simulink model "HeatExchanger"  (Simulink 8.3)
settings: Solver=ode4  StartTime=0.0  StopTime=800  FixedStep=.01  RelTol=1e-3
values from neighbouring files (symbols this model uses):
  delta_t = 0.5    [DoublePlant_STAT.mat]    (also in HeatExchanger_ps.m = 0.1; Initials.mat = 0.25; steady_state_data.mat = 0.1)
libraries: simulink x1
settings Model: Creator=Rhine  LastModifiedBy=wangwenchen
settings OptimizationCC: ExpressionDepthLimit=2147483647
settings DebuggingCC: FcnCallInpInsideContextMsg=UseLocalSettings

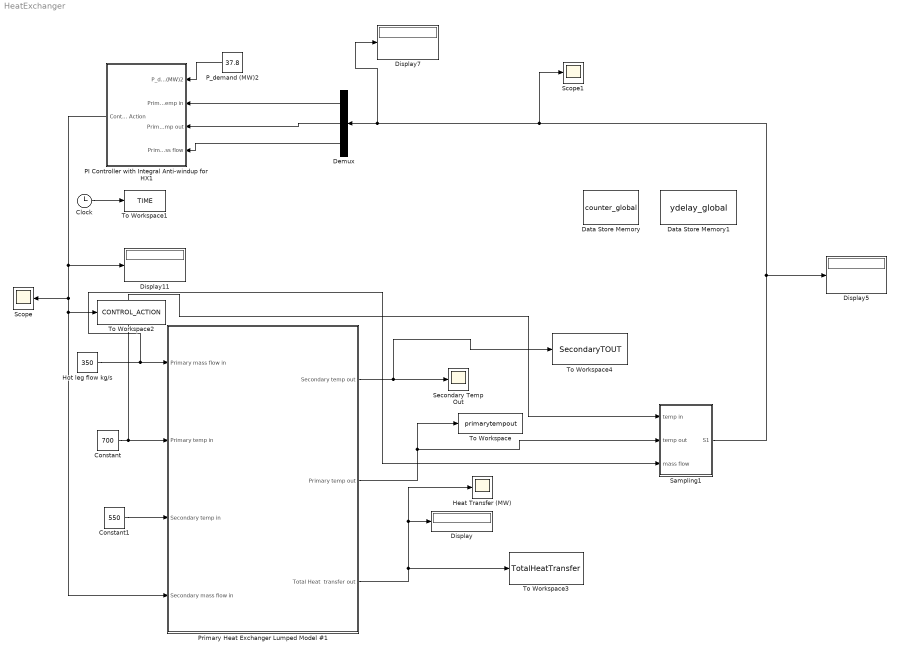
== system HeatExchanger ==
  Clock : Clock
  Constant : Constant  Value=700
  Constant1 : Constant  Value=550
  Data Store Memory : DataStoreMemory  DataStoreName=counter_global  ReadBeforeWriteMsg=warning  WriteAfterWriteMsg=warning  WriteAfterReadMsg=warning  OutDataTypeStr=int32
  Data Store Memory1 : DataStoreMemory  DataStoreName=ydelay_global  ReadBeforeWriteMsg=warning  WriteAfterWriteMsg=warning  WriteAfterReadMsg=warning  InitialValue=ones(10,1)  OutDataTypeStr=int32
  Demux : Demux  Outputs=3
  Display{,5,7,11} (4 alike) : Display
  Heat Transfer (MW) : Scope
      settings: TimeRange=30  YMin=23.3769  YMax=25.8377  SaveName=ScopeData3
  Hot leg flow kg/s : Constant  Value=350
  PI Controller with Integral Anti-windup for HX1 : Subsystem
  P_demand (MW)2 : Constant  Value=37.8
  Primary Heat Exchanger Lumped Model #1 : Subsystem
  Sampling1 : Subsystem
  Scope : Scope
      settings: SaveName=ScopeData2
  Scope1 : Scope
      settings: SaveName=ScopeData5
  Secondary Temp Out : Scope
      settings: YMin=639  YMax=640.4
  To Workspace : ToWorkspace  VariableName=primarytempout  SaveFormat=Timeseries  SampleTime=-1
  To Workspace1 : ToWorkspace  VariableName=TIME  SampleTime=-1
  To Workspace2 : ToWorkspace  VariableName=CONTROL_ACTION  SaveFormat=Timeseries  SampleTime=-1
  To Workspace3 : ToWorkspace  VariableName=TotalHeatTransfer  SaveFormat=Timeseries  SampleTime=-1
  To Workspace4 : ToWorkspace  VariableName=SecondaryTOUT  SaveFormat=Timeseries  SampleTime=-1
  wires:
  Clock/1 -> To Workspace1/1
  Sampling1/1(S1) -> Scope1/1, Display7/1, Demux/1, Display5/1
  P_demand (MW)2/1 -> PI Controller with Integral Anti-windup for HX1/1(P_demand (MW)2)
  Hot leg flow kg/s/1 -> Primary Heat Exchanger Lumped Model #1/1(Primary mass flow in), Sampling1/3(mass flow)
  Constant/1 -> Sampling1/1(temp in), Primary Heat Exchanger Lumped Model #1/2(Primary temp in)
  Constant1/1 -> Primary Heat Exchanger Lumped Model #1/3(Secondary temp in)
  Primary Heat Exchanger Lumped Model #1/2(Primary temp out) -> To Workspace/1, Sampling1/2(temp out)
  Primary Heat Exchanger Lumped Model #1/1(Secondary temp out) -> To Workspace4/1, Secondary Temp Out/1
  Demux/1 -> PI Controller with Integral Anti-windup for HX1/2(Primary temp in)
  Demux/2 -> PI Controller with Integral Anti-windup for HX1/3(Primary temp out)
  Demux/3 -> PI Controller with Integral Anti-windup for HX1/4(Primary mass flow)
  PI Controller with Integral Anti-windup for HX1/1(Control Action) -> Display11/1, Scope/1, Primary Heat Exchanger Lumped Model #1/4(Secondary mass flow in), To Workspace2/1
  Primary Heat Exchanger Lumped Model #1/3("Total Heat  transfer out ") -> Heat Transfer (MW)/1, Display/1, To Workspace3/1

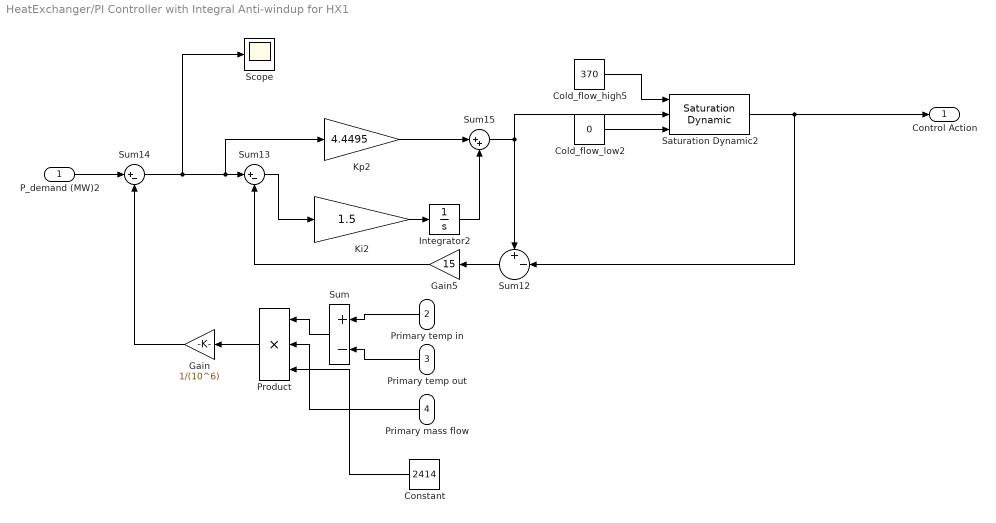
== system HeatExchanger/PI Controller with Integral Anti-windup for HX1 ==
  P_demand (MW)2 : Inport
  Primary temp in : Inport  Port=2
  Primary temp out : Inport  Port=3
  Primary mass flow : Inport  Port=4
  Cold_flow_high5 : Constant  Value=370
  Cold_flow_low2 : Constant  Value=0
  Constant : Constant  Value=2414
  Gain : Gain  Gain=1/(10^6)
  Gain5 : Gain  Gain=15
  Integrator2 : Integrator  InitialCondition=210.3
  Ki2 : Gain  Gain=1.5
  Kp2 : Gain  Gain=4.4495
  Product : Product  Inputs=3
  Saturation Dynamic2 : simulink/Discontinuities/Saturation Dynamic  OutMin=[]  OutMax=[]  OutDataTypeStr=Inherit: Same as second input  OutDataType=fixdt(1, 16)  OutScaling=2^-10  DoSatur=off
  Scope : Scope
      settings: SaveName=ScopeData4
  Sum : Sum  Inputs=+-
  Sum12 : Sum  Inputs=+-|
  Sum13 : Sum  Inputs=|+-
  Sum14 : Sum  Inputs=|+-
  Sum15 : Sum  Inputs=|++
  Control Action : Outport
  wires:
  Product/1 -> Gain/1
  Cold_flow_low2/1 -> Saturation Dynamic2/3
  Cold_flow_high5/1 -> Saturation Dynamic2/1
  Sum14/1 -> Scope/1, Kp2/1, Sum13/1
  P_demand (MW)2/1 -> Sum14/1
  Sum12/1 -> Gain5/1
  Integrator2/1 -> Sum15/2
  Gain5/1 -> Sum13/2
  Sum13/1 -> Ki2/1
  Ki2/1 -> Integrator2/1
  Kp2/1 -> Sum15/1
  Saturation Dynamic2/1 -> Control Action/1, Sum12/2
  Sum15/1 -> Sum12/1, Saturation Dynamic2/2
  Primary temp in/1 -> Sum/1
  Primary temp out/1 -> Sum/2
  Sum/1 -> Product/1
  Primary mass flow/1 -> Product/2
  Constant/1 -> Product/3
  Gain/1 -> Sum14/2

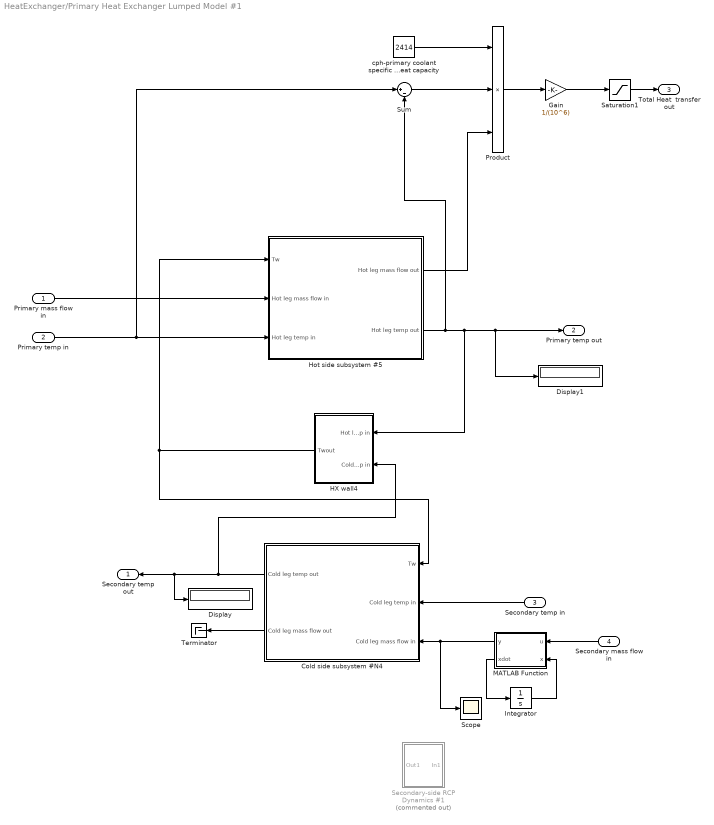
== system HeatExchanger/Primary Heat Exchanger Lumped Model #1 ==
  Primary mass flow in : Inport
  Primary temp in : Inport  Port=2
  Secondary temp in : Inport  Port=3
  Secondary mass flow in : Inport  Port=4
  Cold side subsystem #N4 : Subsystem
  Display : Display
  Display1 : Display
  Gain : Gain  Gain=1/(10^6)
  HX wall4 : Subsystem
  Hot side subsystem #5 : Subsystem
  Integrator : Integrator  InitialCondition=210.3
  MATLAB Function : MATLAB Function  TreatAsAtomicUnit=on
  Product : Product  Inputs=3
  Saturation1 : Saturate  UpperLimit=inf  LowerLimit=0
  Scope : Scope
      settings: SaveName=ScopeData6
  Secondary-side RCP Dynamics #1 : Subsystem  Commented=on
  Sum : Sum  Inputs=|+-
  Terminator : Terminator
  cph-primary coolant specific heat capacity : Constant  Value=2414
  Secondary temp out : Outport
  Primary temp out : Outport  Port=2
  "Total Heat  transfer out " : Outport  Port=3
  wires:
  Cold side subsystem #N4/1(Cold leg temp out) -> Display/1, Secondary temp out/1, HX wall4/2(Cold leg temp in)
  Cold side subsystem #N4/2(Cold leg mass flow out) -> Terminator/1
  Primary mass flow in/1 -> Hot side subsystem #5/2(Hot leg mass flow in)
  Primary temp in/1 -> Hot side subsystem #5/3(Hot leg temp in), Sum/1
  Secondary mass flow in/1 -> MATLAB Function/1(u)
  Secondary temp in/1 -> Cold side subsystem #N4/2(Cold leg temp in)
  HX wall4/1(Twout) -> Cold side subsystem #N4/1(Tw), Hot side subsystem #5/1(Tw)
  Hot side subsystem #5/1(Hot leg mass flow out) -> Product/3
  Hot side subsystem #5/2(Hot leg temp out) -> HX wall4/1(Hot leg temp in), Display1/1, Primary temp out/1, Sum/2
  cph-primary coolant specific heat capacity/1 -> Product/1
  Sum/1 -> Product/2
  Product/1 -> Gain/1
  Gain/1 -> Saturation1/1
  MATLAB Function/1(y) -> Cold side subsystem #N4/3(Cold leg mass flow in), Scope/1
  Saturation1/1 -> "Total Heat  transfer out "/1
  MATLAB Function/2(xdot) -> Integrator/1
  Integrator/1 -> MATLAB Function/2(x)

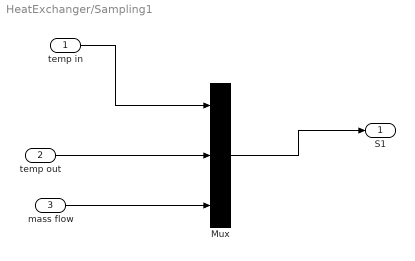
== system HeatExchanger/Sampling1 ==
  temp in : Inport
  temp out : Inport  Port=2
  mass flow : Inport  Port=3
  Mux : Mux  Inputs=3
  S1 : Outport
  wires:
  temp in/1 -> Mux/1
  temp out/1 -> Mux/2
  mass flow/1 -> Mux/3
  Mux/1 -> S1/1

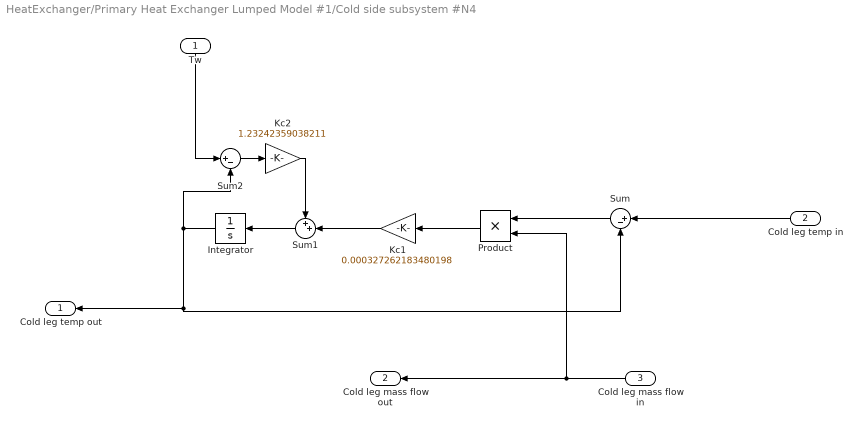
== system HeatExchanger/Primary Heat Exchanger Lumped Model #1/Cold side subsystem #N4 ==
  Tw : Inport
  Cold leg temp in : Inport  Port=2
  Cold leg mass flow in : Inport  Port=3
  Integrator : Integrator  InitialCondition=644.5
  Kc1 : Gain  Gain=0.000327262183480198
  Kc2 : Gain  Gain=1.23242359038211
  Product : Product
  Sum : Sum  Inputs=|+-
  Sum1 : Sum  Inputs=++|
  Sum2 : Sum  Inputs=|+-
  Cold leg temp out : Outport
  Cold leg mass flow out : Outport  Port=2
  wires:
  Cold leg temp in/1 -> Sum/1
  Integrator/1 -> Sum/2, Cold leg temp out/1, Sum2/2
  Sum2/1 -> Kc2/1
  Sum/1 -> Product/1
  Kc2/1 -> Sum1/1
  Sum1/1 -> Integrator/1
  Cold leg mass flow in/1 -> Cold leg mass flow out/1, Product/2
  Product/1 -> Kc1/1
  Kc1/1 -> Sum1/2
  Tw/1 -> Sum2/1

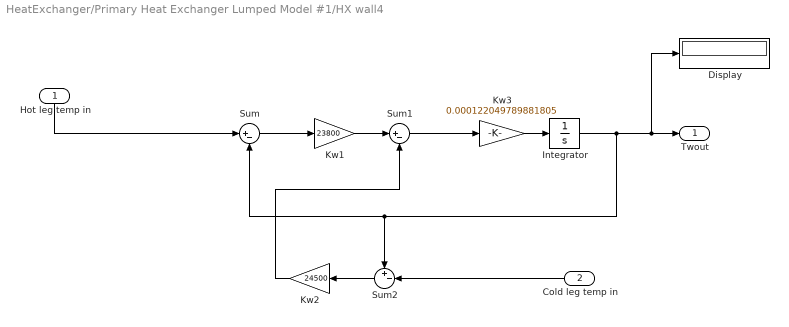
== system HeatExchanger/Primary Heat Exchanger Lumped Model #1/HX wall4 ==
  Hot leg temp in : Inport
  Cold leg temp in : Inport  Port=2
  Display : Display
  Integrator : Integrator  InitialCondition=649.8
  Kw1 : Gain  Gain=23800
  Kw2 : Gain  Gain=24500
  Kw3 : Gain  Gain=0.000122049789881805
  Sum : Sum  Inputs=|+-
  Sum1 : Sum  Inputs=|+-
  Sum2 : Sum  Inputs=+-|
  Twout : Outport
  wires:
  Sum2/1 -> Kw2/1
  Hot leg temp in/1 -> Sum/1
  Sum1/1 -> Kw3/1
  Cold leg temp in/1 -> Sum2/2
  Sum/1 -> Kw1/1
  Kw1/1 -> Sum1/1
  Kw3/1 -> Integrator/1
  Integrator/1 -> Display/1, Twout/1, Sum2/1, Sum/2
  Kw2/1 -> Sum1/2

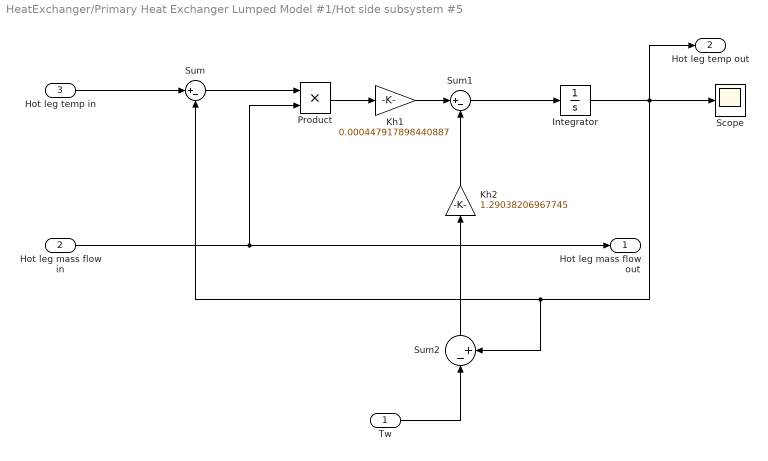
== system HeatExchanger/Primary Heat Exchanger Lumped Model #1/Hot side subsystem #5 ==
  Tw : Inport
  Hot leg mass flow in : Inport  Port=2
  Hot leg temp in : Inport  Port=3
  Integrator : Integrator  InitialCondition=655.3
  Kh1 : Gain  Gain=0.000447917898440887
  Kh2 : Gain  Gain=1.29038206967745
  Product : Product
  Scope : Scope
  Sum : Sum  Inputs=|+-
  Sum1 : Sum  Inputs=|+-
  Sum2 : Sum  Inputs=|-+
  Hot leg mass flow out : Outport
  Hot leg temp out : Outport  Port=2
  wires:
  Product/1 -> Kh1/1
  Kh1/1 -> Sum1/1
  Sum1/1 -> Integrator/1
  Sum2/1 -> Kh2/1
  Kh2/1 -> Sum1/2
  Tw/1 -> Sum2/1
  Hot leg temp in/1 -> Sum/1
  Hot leg mass flow in/1 -> Hot leg mass flow out/1, Product/2
  Sum/1 -> Product/1
  Integrator/1 -> Hot leg temp out/1, Scope/1, Sum2/2, Sum/2

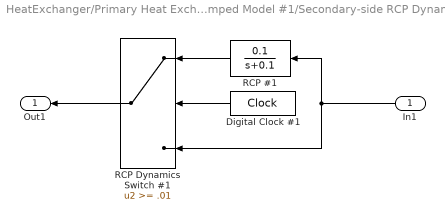
== system HeatExchanger/Primary Heat Exchanger Lumped Model #1/Secondary-side RCP Dynamics #1 ==
  In1 : Inport
  Digital Clock #1 : DigitalClock  SampleTime=delta_t
  RCP #1 : TransferFcn  Numerator=[0.1]  Denominator=[1 0.1]
  RCP Dynamics Switch #1 : Switch  Threshold=.01
  Out1 : Outport
  wires:
  In1/1 -> RCP #1/1, RCP Dynamics Switch #1/3
  Digital Clock #1/1 -> RCP Dynamics Switch #1/2
  RCP #1/1 -> RCP Dynamics Switch #1/1
  RCP Dynamics Switch #1/1 -> Out1/1

== matlab function Primary Heat Exchanger Lumped Model #1/MATLAB Function ==
  data: u input double; y output double; x input double; xdot output double
function [y,xdot] = pump(u,x)
%#codegen

if u<0
    u=0;
else
end

xdot = -0.1*x + 0.1*u;

y = x;
